simulink model "simfile"  (R2024a)
settings: Solver=VariableStepAuto  StartTime=0.0  StopTime=10.0  RelTol=1e-3
values from neighbouring files (symbols this model uses):
  U = input("enter the value of U: ")    [mscript.m]
libraries: simulink x1
settings Model: Creator=admin  LastModifiedBy=admin

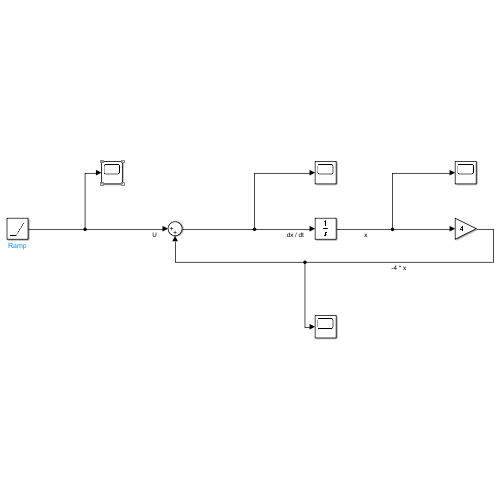
[thumbnail: Simulink's stored preview of the top-level diagram]
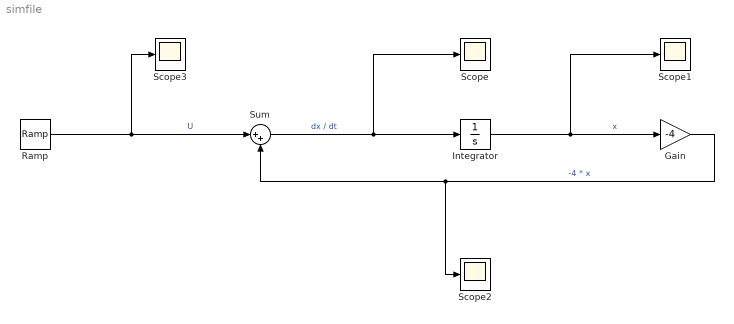
== system simfile ==
  Gain : Gain  Gain=-4
  Integrator : Integrator
  Ramp : simulink/Sources/Ramp  slope=U  start=0  InitialOutput=0
  Scope{,1..3} (4 alike) : Scope
  Sum : Sum  Inputs=|++
  wires:
  Sum/1 -> Scope/1, Integrator/1  "dx / dt"
  Integrator/1 -> Scope1/1, Gain/1  "x"
  Gain/1 -> Scope2/1, Sum/2  "-4 * x"
  Ramp/1 -> Sum/1, Scope3/1  "U"
